simulink model "SensorErrorModel"  (R2015b)
settings: Solver=VariableStepAuto  StartTime=0.0  StopTime=10.0  RelTol=1e-3
settings Model: Creator=jeremie  LastModifiedBy=jeremie

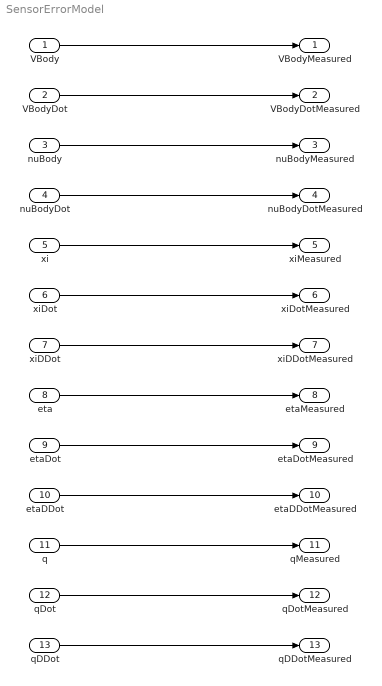
== system SensorErrorModel ==
  VBody : Inport  PortDimensions=3
  VBodyDot : Inport  Port=2  PortDimensions=3
  nuBody : Inport  Port=3  PortDimensions=3
  nuBodyDot : Inport  Port=4  PortDimensions=3
  xi : Inport  Port=5  PortDimensions=3
  xiDot : Inport  Port=6  PortDimensions=3
  xiDDot : Inport  Port=7  PortDimensions=3
  eta : Inport  Port=8  PortDimensions=3
  etaDot : Inport  Port=9  PortDimensions=3
  etaDDot : Inport  Port=10  PortDimensions=3
  q : Inport  Port=11  PortDimensions=4
  qDot : Inport  Port=12  PortDimensions=4
  qDDot : Inport  Port=13  PortDimensions=4
  VBodyMeasured : Outport
  VBodyDotMeasured : Outport  Port=2
  nuBodyMeasured : Outport  Port=3
  nuBodyDotMeasured : Outport  Port=4
  xiMeasured : Outport  Port=5
  xiDotMeasured : Outport  Port=6
  xiDDotMeasured : Outport  Port=7
  etaMeasured : Outport  Port=8
  etaDotMeasured : Outport  Port=9
  etaDDotMeasured : Outport  Port=10
  qMeasured : Outport  Port=11
  qDotMeasured : Outport  Port=12
  qDDotMeasured : Outport  Port=13
  wires:
  VBody/1 -> VBodyMeasured/1
  VBodyDot/1 -> VBodyDotMeasured/1
  nuBody/1 -> nuBodyMeasured/1
  nuBodyDot/1 -> nuBodyDotMeasured/1
  xi/1 -> xiMeasured/1
  xiDot/1 -> xiDotMeasured/1
  xiDDot/1 -> xiDDotMeasured/1
  eta/1 -> etaMeasured/1
  etaDot/1 -> etaDotMeasured/1
  etaDDot/1 -> etaDDotMeasured/1
  q/1 -> qMeasured/1
  qDot/1 -> qDotMeasured/1
  qDDot/1 -> qDDotMeasured/1
